simulink model "trajectory_generator"  (R2019b)
settings: Solver=ode45  StartTime=0.0  StopTime=10  MaxStep=0.01  RelTol=1e-3
values from neighbouring files (symbols this model uses):
  D = [eye(6)*0; eye(6)]    [trajLine.m]
  qq = ikine6s(p560,TTc)    [trajCircle.m]    (also in trajLine.m = ikine6s(p560,TTl))
undefined symbols (not defined in the file or in its folder): transl
libraries: roblocks x30, dspmtrx3 x3
settings Model: Creator=sarim  LastModifiedBy=sarim

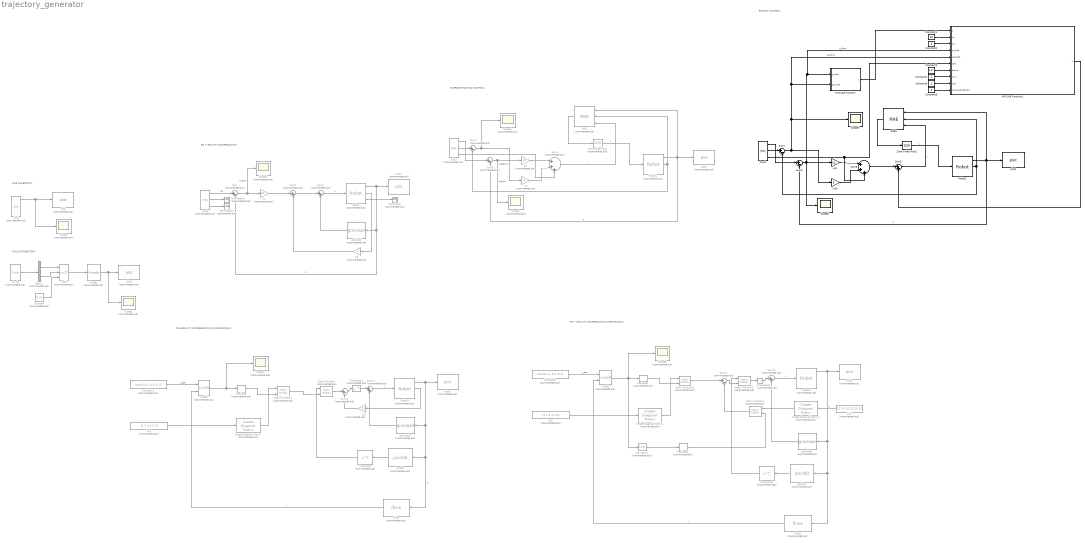
== system trajectory_generator ==
  note: LINE TRAJECTORY
  note: CIRCLE TRAJECTORY
  note: PD + GRAVITY COMPENSATION
  note: INVERSE DYNAMICS CONTROL
  note: ROBUST CONTROL
  note: PD+GRAVITY COMPENSATION IN WORKSPACE 1
  note: PD + GRAVITY COMPENSATION WORKSPACE 2
  Circle : roblocks/Toolbox/Circle  Commented=on  radius=radius  freq=0.2
  Constant : Constant  Commented=on  Value=0.25
  Constant1 : Constant  Value=10
  Constant2 : Constant  Value=3
  Constant3 : Constant  Value=0.01
  Constant4 : Constant
  Constant5 : Constant
  Constant6 : Constant  Value=2
  Constant7 : Constant  Commented=on  Value=transl(0.4, 0.5, 0.2)
  Constant8 : Constant  Commented=on  Value=transl(0.4, 0.5, 0.2)
  Create Diagonal Matrix : dspmtrx3/Create Diagonal Matrix  Commented=on
      settings: SourceProductName=DSP System Toolbox  SourceProductBaseCode=DS
  Create Diagonal Matrix1 : dspmtrx3/Create Diagonal Matrix  Commented=on
      settings: SourceProductName=DSP System Toolbox  SourceProductBaseCode=DS
  Create Diagonal Matrix2 : dspmtrx3/Create Diagonal Matrix  Commented=on
      settings: SourceProductName=DSP System Toolbox  SourceProductBaseCode=DS
  Demux : Demux  Commented=on  Outputs=2
  Derivative : Derivative  Commented=on
  KD : Gain  Commented=on  Gain=3
  KDD : Gain  Gain=3
  KP : Gain  Commented=on  Gain=10
  KPP : Gain  Gain=10
  Kd : Gain  Commented=on  Gain=3
  Kd1 : Gain  Commented=on  Gain=10
  "Kd2 " : Constant  Commented=on  Value=[10 10 10 10 10 10]
  Kp : Gain  Commented=on  Gain=10
  Kp1 : Constant  Commented=on  Value=[3 3 3 3 3 3]
  Kp2 : Constant  Commented=on  Value=[3 3 3 3 3 3]
  MATLAB Function : MATLAB Function  TreatAsAtomicUnit=on
  MATLAB Function1 : MATLAB Function  TreatAsAtomicUnit=on
  Matrix Multiply{,1..4} (5 alike) : Product  Commented=on  Multiplication=Matrix(*)
  RNE : roblocks/Arm/RNE  Commented=on  robot=p560Uncnofriction  grav=[0 0 9.81]
  RNE1 : roblocks/Arm/RNE  robot=p560Uncnofriction  grav=[0 0 9.81]
  Reshape : Reshape  Commented=on  OutputDimensionality=Column vector (2-D)
  Reshape1 : Reshape  Commented=on  OutputDimensionality=Column vector (2-D)
  Reshape2 : Reshape  Commented=on  OutputDimensionality=Column vector (2-D)
  Robot{,1,3..4} (4 alike) : roblocks/Arm/Robot  Commented=on  robot=pumanofriction  q0=[0 0 0 0 0 0]
  Robot2 : roblocks/Arm/Robot  robot=pumanofriction  q0=[0 0 0 0 0 0]
  Scope{,1..4,7..8} (7 alike) : Scope  Commented=on
  Scope5 : Scope
  Scope6 : Scope
  Sum{,1,3..4,10..11} (6 alike) : Sum  Commented=on  Inputs=|+-
  Sum12 : Sum  Commented=on  Inputs=|++
  Sum13 : Sum  Commented=on  Inputs=|++
  Sum2 : Sum  Commented=on  Inputs=|++
  Sum5 : Sum  Commented=on  Inputs=|+++
  Sum6 : Sum  Inputs=|+-
  Sum7 : Sum  Inputs=|+-
  Sum8 : Sum  Inputs=|+++
  Sum9 : Sum  Inputs=|++
  Terminator : Terminator  Commented=on
  Terminator1 : Terminator  Commented=on
  Terminator2 : Terminator  Commented=on
  Transpose{,1..3} (4 alike) : Math  Commented=on  Operator=transpose  SignedPower=off  SaturateOnIntegerOverflow=on
  Zero-Order Hold : ZeroOrderHold  Commented=on  SampleTime=-1
  Zero-Order Hold1 : ZeroOrderHold  SampleTime=-1
  fkine : roblocks/Arm/fkine  Commented=on  robot=pumanofriction
  fkine1 : roblocks/Arm/fkine  Commented=on  robot=pumanofriction
  gravload : roblocks/Arm/gravload  Commented=on  robot=pumanofriction
  gravload1 : roblocks/Arm/gravload  Commented=on  robot=pumanofriction
  gravload2 : roblocks/Arm/gravload  Commented=on  robot=pumanofriction
  ikine6s : roblocks/Arm/ikine6s  Commented=on  robot=p560  conf='luf'
  "jacob0 " : roblocks/Arm/jacob0   Commented=on  robot=pumanofriction
  jacob0 1 : roblocks/Arm/jacob0   Commented=on  robot=pumanofriction
  jtraj : roblocks/Toolbox/jtraj  Commented=on  q0=qq(1,:)  qf=qq(end,:)  tmax=tfin  ts=0.01
  jtraj1 : roblocks/Toolbox/jtraj  Commented=on  q0=qq(1,:)  qf=qq(end,:)  tmax=10  ts=0.1
  jtraj2 : roblocks/Toolbox/jtraj  Commented=on  q0=qq(1,:)  qf=qq(end,:)  tmax=10  ts=0.02
  jtraj3 : roblocks/Toolbox/jtraj  q0=qq(1,:)  qf=qq(end,:)  tmax=10  ts=0.1
  plot{,1..3,5..6} (6 alike) : roblocks/Arm/plot  Commented=on  robot=p560  fps=5  holdplot=on
  plot4 : roblocks/Arm/plot  robot=p560  fps=5  holdplot=on
  tr2diff : roblocks/Toolbox/tr2diff  Commented=on  robot=pumanofriction
  tr2diff1 : roblocks/Toolbox/tr2diff  Commented=on  robot=pumanofriction
  xyz2T : roblocks/Toolbox/xyz2T  Commented=on
  wires:
  jtraj/1 -> Scope/1, plot/1
  Circle/1 -> Demux/1
  Demux/1 -> xyz2T/1
  Demux/2 -> xyz2T/2
  xyz2T/1 -> ikine6s/1
  ikine6s/1 -> Scope1/1, plot1/1
  Constant/1 -> xyz2T/3
  jtraj1/1 -> Sum/1  "qd"
  Sum/1 -> Scope2/1, Kp/1  "q_error"
  Kp/1 -> Sum1/1
  Sum1/1 -> Sum2/1
  gravload/1 -> Sum2/2
  Robot/2 -> Kd/1
  Kd/1 -> Sum1/2
  Robot/1 -> Sum/2, gravload/1, plot2/1  "q"
  Robot/3 -> Terminator/1
  jtraj1/2 -> Terminator1/1
  jtraj1/3 -> Terminator2/1
  Sum2/1 -> Robot/1  "u"
  jtraj2/1 -> Sum3/1
  Sum3/1 -> Scope4/1, KP/1  "q_Error"
  Sum4/1 -> Scope3/1, KD/1  "qd_Error"
  jtraj2/2 -> Sum4/1
  KP/1 -> Sum5/1
  KD/1 -> Sum5/2
  jtraj2/3 -> Sum5/3
  Robot1/1 -> plot3/1, Sum3/2, RNE/1  "q"
  Robot1/2 -> RNE/2, Sum4/2
  RNE/1 -> Zero-Order Hold/1
  Sum5/1 -> RNE/3  "y"
  Zero-Order Hold/1 -> Robot1/1  "u"
  Robot2/1 -> plot4/1, Sum6/2, RNE1/1  "q"
  KPP/1 -> Sum8/1
  RNE1/1 -> Zero-Order Hold1/1
  jtraj3/2 -> Sum7/1
  Robot2/2 -> RNE1/2, Sum7/2
  KDD/1 -> Sum8/2
  Zero-Order Hold1/1 -> Robot2/1  "u"
  Sum6/1 -> MATLAB Function1/4(q_tilde), MATLAB Function/1(q_tilde), Scope6/1, KPP/1  "q_Error"
  jtraj3/1 -> Sum6/1
  Sum7/1 -> MATLAB Function1/5(qd_tilde), MATLAB Function/2(qd_tilde), Scope5/1, KDD/1  "qd_Error"
  jtraj3/3 -> MATLAB Function1/6(qdd), Sum8/3
  MATLAB Function/1(z) -> MATLAB Function1/1(z)
  Constant1/1 -> MATLAB Function1/2(Kp)
  Constant2/1 -> MATLAB Function1/3(Kd)
  Constant3/1 -> MATLAB Function1/7(alpha)
  Constant4/1 -> MATLAB Function1/8(M_M)
  Constant5/1 -> MATLAB Function1/9(N_M)
  Sum8/1 -> Sum9/1
  MATLAB Function1/1(w) -> Sum9/2
  Sum9/1 -> RNE1/3  "y"
  Constant6/1 -> MATLAB Function1/10(sliding_threshold)
  Sum12/1 -> Robot3/1  "u"
  Robot3/1 -> "jacob0 "/1, fkine/1, gravload1/1, plot5/1  "q"
  fkine/1 -> tr2diff/2  "x"
  "jacob0 "/1 -> Transpose/1
  Constant7/1 -> tr2diff/1  "x_star"
  tr2diff/1 -> Reshape/1, Scope7/1
  Robot3/2 -> Kd1/1
  Matrix Multiply/1 -> Sum10/1
  gravload1/1 -> Sum12/2
  Kd1/1 -> Sum10/2
  Kp1/1 -> Create Diagonal Matrix/1
  Create Diagonal Matrix/1 -> Matrix Multiply1/1
  Reshape/1 -> Matrix Multiply1/2
  Transpose/1 -> Matrix Multiply/1
  Matrix Multiply1/1 -> Matrix Multiply/2
  "Kd2 "/1 -> Create Diagonal Matrix2/1
  tr2diff1/1 -> Derivative/1, Reshape1/1, Scope8/1
  Transpose2/1 -> Matrix Multiply2/1
  Kp2/1 -> Create Diagonal Matrix1/1
  Sum13/1 -> Robot4/1  "u"
  fkine1/1 -> tr2diff1/2  "x"
  Transpose3/1 -> Sum13/1
  Create Diagonal Matrix2/1 -> Matrix Multiply4/1
  Sum11/1 -> Matrix Multiply2/2
  gravload2/1 -> Sum13/2
  Constant8/1 -> tr2diff1/1  "x_star"
  Create Diagonal Matrix1/1 -> Matrix Multiply3/1
  jacob0 1/1 -> Transpose2/1
  Matrix Multiply2/1 -> Transpose3/1
  Matrix Multiply4/1 -> Sum11/2
  Robot4/1 -> jacob0 1/1, fkine1/1, gravload2/1, plot6/1  "q"
  Matrix Multiply3/1 -> Sum11/1
  Reshape1/1 -> Matrix Multiply3/2
  Sum10/1 -> Transpose1/1
  Transpose1/1 -> Sum12/1
  Derivative/1 -> Reshape2/1
  Reshape2/1 -> Matrix Multiply4/2

== matlab function trajectory_generator/MATLAB Function1 ==
  data: z input; w output; Kp input; Kd input; q_tilde input; qd_tilde input; qdd input; alpha input; M_M input; N_M input; sliding_threshold input
function w = calc_unc(z, Kp, Kd, q_tilde, qd_tilde, qdd, alpha, M_M, N_M, sliding_threshold)
    K = [eye(6)*Kp eye(6)*Kd];
    epsilon = [q_tilde; qd_tilde];
    Q_M = max(abs(qdd)) + 0.1;
    rho = (1/(1-alpha))*(alpha*Q_M + alpha*norm(K)*norm(epsilon) + M_M*N_M);
    z_unit_vector = z/norm(z);
    if norm(z) >= sliding_threshold
        w = rho * z_unit_vector;
    else
        w = rho * z * (1/sliding_threshold);
    end
end

== matlab function trajectory_generator/MATLAB Function ==
  settings: updateMethod=DISCRETE
  data: q_tilde input; z output; qd_tilde input
function z = calc_z(q_tilde, qd_tilde)
D = [eye(6)*0; eye(6)];
matrixSize = 12;
while true
  A = randi ([1 5], matrixSize, matrixSize);
  if rank (A) == matrixSize; break ; end % will be true nearly all the time    
end
Q = A' * A;
epsilon = [q_tilde; qd_tilde];
z = transpose(D) * 100 * Q * epsilon;
end
